simulink model "row_stanu_model"  (R2015a)
settings: Solver=ode45  StartTime=0.0  StopTime=czas_sym  MaxStep=tmax  RelTol=1e-3
values from neighbouring files (symbols this model uses):
  A = [ (Kg^2 - MTw*Kg)/m1,              (Kg*Kw)/m1;          (Kg*Kw)/m2,     -(- Kw^2 + MTw*Kw + Ks*MTw)/m2]    [row_stanu.m]    (also in ss_tf_support.m)
  B = [ 1/Cvg,      (Kg*P)/m1;               0,          (Ks*MTw + Kw*P)/m2]    [row_stanu.m]    (also in ss_tf_support.m)
  C = [1 , 0; 0, 1; Kg/MTw, Kw/MTw]    [row_stanu.m]    (also in ss_tf_support.m)
  D = [0 , 0; 0, 0; 0, P/MTw]    [row_stanu.m]    (also in ss_tf_support.m)
  dQg = QgN*0.1    [dokladny.m]    (also in kupfmuller.m; row_stanu.m; ss_tf.m; transmitancje.m = QgN*0.0)
  dTzew = 0    [dokladny.m]    (also in kupfmuller.m; row_stanu.m; ss_tf.m = 2; transmitancje.m = 2)
  Qg0 = wektor_Qg0(i)    [char_czestotliwosciowe.m]    (also in char_statyczne.m = [0.7*QgN : 0.1*QgN : (1.3*QgN)]; dokladny.m; kupfmuller.m; row_stanu.m)
  t0 = 40000    [dokladny.m]    (also in kupfmuller.m; row_stanu.m; transmitancje.m)
  Tzew0 = wektor_Tzew0(i)    [char_czestotliwosciowe.m]    (also in char_statyczne.m = [0.7*TzewN : 0.1*TzewN : 1.3*TzewN]; dokladny.m; kupfmuller.m; row_stanu.m)
  x0 = (-A^-1) * (B*u0)    [row_stanu.m]    (also in ss_tf_support.m)
settings Model: Creator=Prezes  LastModifiedBy=Prezes

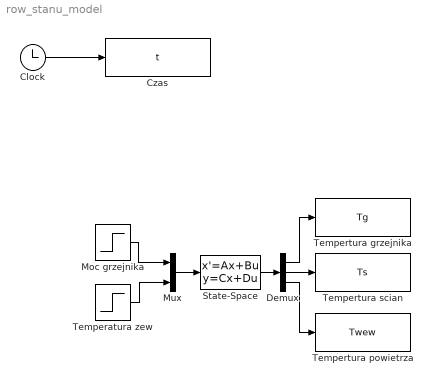
== system row_stanu_model ==
  Clock : Clock
  Czas : ToWorkspace  VariableName=t  SampleTime=-1
      settings: Save2DSignal=2-D array (concatenate along first dimension)
  Demux : Demux  Outputs=3
  Moc grzejnika : Step  Time=t0  Before=Qg0  After=Qg0 + dQg  SampleTime=0
  Mux : Mux  Inputs=2
  State-Space : StateSpace  A=A  B=B  C=C  D=D  X0=x0
  Temperatura zew : Step  Time=t0  Before=Tzew0  After=Tzew0+ dTzew  SampleTime=0
  Tempertura grzejnika : ToWorkspace  VariableName=Tg  SampleTime=-1
      settings: Save2DSignal=2-D array (concatenate along first dimension)
  Tempertura powietrza : ToWorkspace  VariableName=Twew  SampleTime=-1
      settings: Save2DSignal=2-D array (concatenate along first dimension)
  Tempertura scian : ToWorkspace  VariableName=Ts  SampleTime=-1
      settings: Save2DSignal=2-D array (concatenate along first dimension)
  wires:
  Clock/1 -> Czas/1
  Temperatura zew/1 -> Mux/2
  Mux/1 -> State-Space/1
  State-Space/1 -> Demux/1
  Moc grzejnika/1 -> Mux/1
  Demux/1 -> Tempertura grzejnika/1
  Demux/2 -> Tempertura scian/1
  Demux/3 -> Tempertura powietrza/1
